simulink library "enm"  (R2022a)
settings: Solver=VariableStepAuto  StartTime=0.0  StopTime=10.0  RelTol=1e-3
undefined symbols (not defined in the file): raptor_xcp_function
libraries: Raptor_lib x7, simulink x2, slpidlib x2
settings Model: Creator=saumilj  LastModifiedBy=saumi

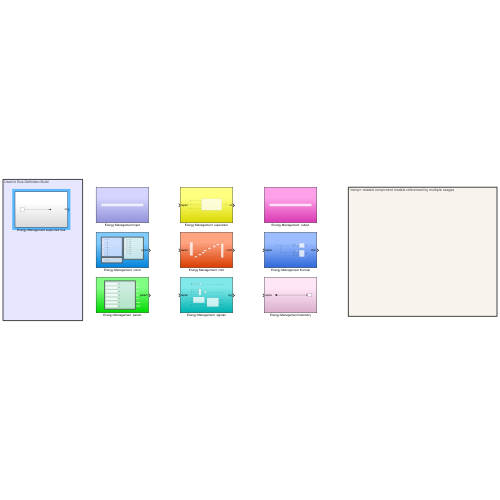
[thumbnail: Simulink's stored preview of the top-level diagram]
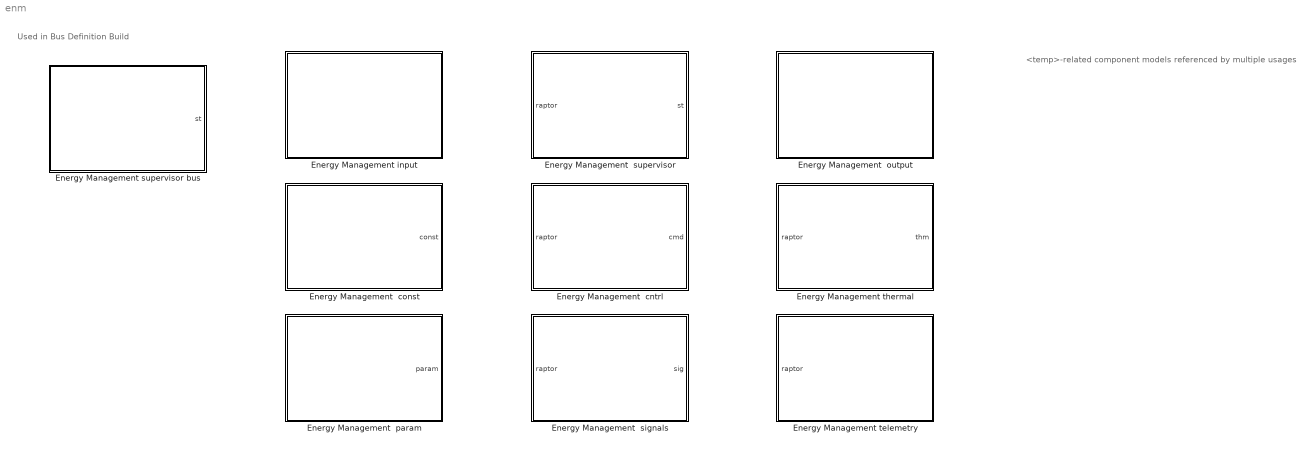
== system enm ==
  note: <temp>-related component models referenced by multiple usages
  note: Used in Bus Definition Build
  Energy Management  cntrl : Subsystem
  Energy Management  const : Subsystem
  Energy Management  output : Subsystem
  Energy Management  param : Subsystem
  Energy Management  signals : Subsystem
  Energy Management  supervisor : Subsystem
  Energy Management input : Subsystem
  Energy Management supervisor bus : Subsystem
  Energy Management telemetry : Subsystem
  Energy Management thermal : Subsystem

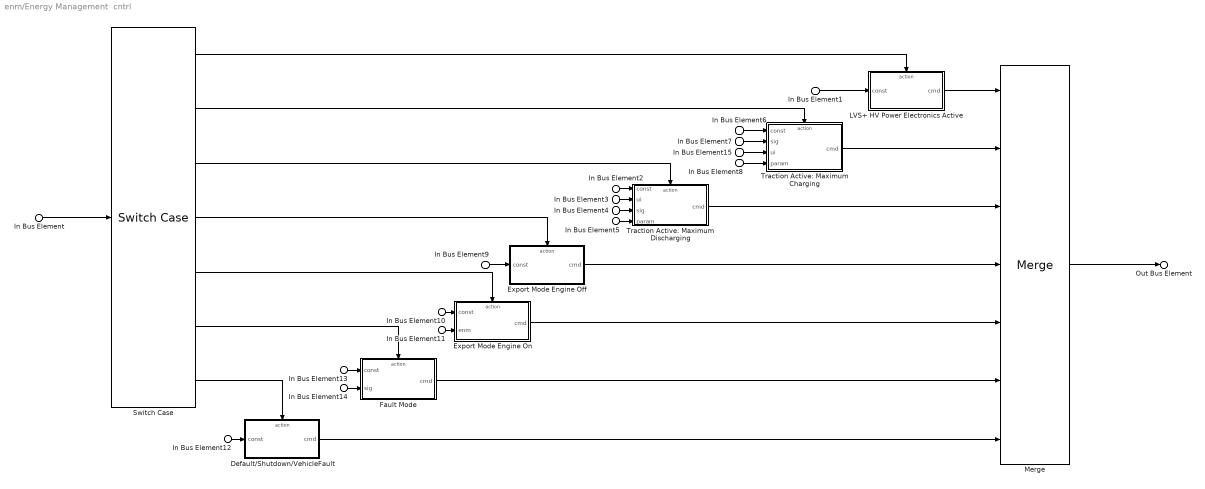
== system enm/Energy Management  cntrl ==
  In Bus Element11 : Inport  PortName=raptor  Element=enm
  In Bus Element : Inport  PortName=raptor  Element=enm.st
  In Bus Element{1..2,6,9..10,12..13} (7 alike) : Inport  PortName=raptor  Element=enm.const
  In Bus Element4 : Inport  PortName=raptor  Element=enm.sig
  In Bus Element7 : Inport  PortName=raptor  Element=enm.sig
  In Bus Element14 : Inport  PortName=raptor  Element=enm.sig
  In Bus Element8 : Inport  PortName=raptor  Element=enm.param
  In Bus Element5 : Inport  PortName=raptor  Element=enm.param
  In Bus Element3 : Inport  PortName=raptor  Element=ui
  In Bus Element15 : Inport  PortName=raptor  Element=ui
  Default/Shutdown/VehicleFault : Subsystem  TreatAsAtomicUnit=on
  Export Mode Engine Off : Subsystem  TreatAsAtomicUnit=on
  Export Mode Engine On : Subsystem  TreatAsAtomicUnit=on
  Fault Mode : Subsystem  TreatAsAtomicUnit=on
  LVS+ HV Power Electronics Active : Subsystem  TreatAsAtomicUnit=on
  Merge : Merge  Inputs=7
  Switch Case : SwitchCase  CaseConditions={1,2,3,4,5,6}
  Traction Active: Maximum Charging : Subsystem  TreatAsAtomicUnit=on
  Traction Active: Maximum Discharging : Subsystem  TreatAsAtomicUnit=on
  Out Bus Element : Outport  PortName=cmd
  wires:
  In Bus Element/1 -> Switch Case/1
  Merge/1 -> Out Bus Element/1
  Switch Case/7 -> Default/Shutdown/VehicleFault/Action
  LVS+ HV Power Electronics Active/1(cmd) -> Merge/1
  Traction Active: Maximum Charging/1(cmd) -> Merge/2
  Traction Active: Maximum Discharging/1(cmd) -> Merge/3
  Export Mode Engine Off/1(cmd) -> Merge/4
  Export Mode Engine On/1(cmd) -> Merge/5
  Fault Mode/1(cmd) -> Merge/6
  Default/Shutdown/VehicleFault/1(cmd) -> Merge/7
  Switch Case/6 -> Fault Mode/Action
  Switch Case/5 -> Export Mode Engine On/Action
  Switch Case/4 -> Export Mode Engine Off/Action
  Switch Case/3 -> Traction Active: Maximum Discharging/Action
  Switch Case/2 -> Traction Active: Maximum Charging/Action
  Switch Case/1 -> LVS+ HV Power Electronics Active/Action
  In Bus Element1/1 -> LVS+ HV Power Electronics Active/1(const)
  In Bus Element2/1 -> Traction Active: Maximum Discharging/1(const)
  In Bus Element3/1 -> Traction Active: Maximum Discharging/2(ui)
  In Bus Element4/1 -> Traction Active: Maximum Discharging/3(sig)
  In Bus Element5/1 -> Traction Active: Maximum Discharging/4(param)
  In Bus Element6/1 -> Traction Active: Maximum Charging/1(const)
  In Bus Element7/1 -> Traction Active: Maximum Charging/2(sig)
  In Bus Element8/1 -> Traction Active: Maximum Charging/4(param)
  In Bus Element9/1 -> Export Mode Engine Off/1(const)
  In Bus Element10/1 -> Export Mode Engine On/1(const)
  In Bus Element11/1 -> Export Mode Engine On/2(enm)
  In Bus Element12/1 -> Default/Shutdown/VehicleFault/1(const)
  In Bus Element13/1 -> Fault Mode/1(const)
  In Bus Element14/1 -> Fault Mode/2(sig)
  In Bus Element15/1 -> Traction Active: Maximum Charging/3(ui)

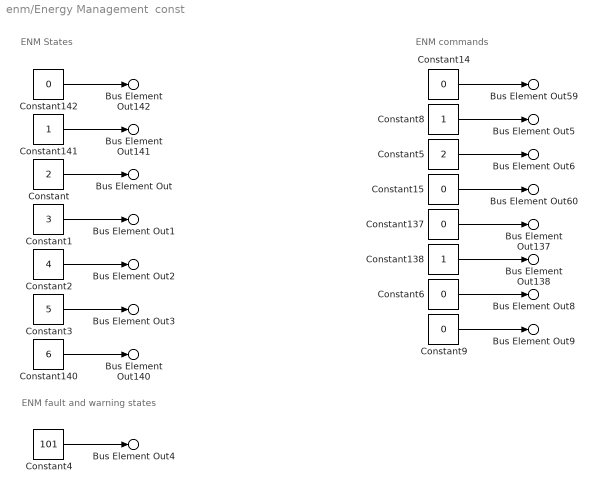
== system enm/Energy Management  const ==
  note: ENM commands
  note: ENM fault and warning states
  note: ENM States
  Constant : Constant  Value=2
  Constant1 : Constant  Value=3
  Constant{6,9,14..15,137,142} (6 alike) : Constant  Value=0
  Constant138 : Constant
  Constant140 : Constant  Value=6
  Constant141 : Constant
  Constant2 : Constant  Value=4
  Constant3 : Constant  Value=5
  Constant4 : Constant  Value=101
  Constant5 : Constant  Value=2
  Constant8 : Constant
  Bus Element Out : Outport  PortName=const  Element=ENM_2_TRACTION_ACTIVE_MAX_CHARGING
  Bus Element Out1 : Outport  PortName=const  Element=ENM_3_TRACTION_ACTIVE_MAX_DISCHARGING
  Bus Element Out2 : Outport  PortName=const  Element=ENM_4_EXPORT_ENG_OFF
  Bus Element Out3 : Outport  PortName=const  Element=ENM_5_EXPORT_ENG_ON
  Bus Element Out59 : Outport  PortName=const  Element=ENM_0_ENG_OFF
  Bus Element Out60 : Outport  PortName=const  Element=ENM_0_ENG_ZERO_POWER_DEMAND
  Bus Element Out137 : Outport  PortName=const  Element=ENM_0_TRAC_REGEN_DISABLE
  Bus Element Out138 : Outport  PortName=const  Element=ENM_1_TRAC_REGEN_ENABLE
  Bus Element Out140 : Outport  PortName=const  Element=ENM_10_SHUTDOWN
  Bus Element Out141 : Outport  PortName=const  Element=ENM_1_IDLE
  Bus Element Out142 : Outport  PortName=const  Element=ENM_0_DEFAULT
  Bus Element Out4 : Outport  PortName=const  Element=ENM_101_REDUCED_POWER
  Bus Element Out5 : Outport  PortName=const  Element=ENM_1_ENG_IDLE
  Bus Element Out6 : Outport  PortName=const  Element=ENM_2_ENG_ON
  Bus Element Out8 : Outport  PortName=const  Element=ENM_0_TRAC_ZERO_SUM_MAX_TQ
  Bus Element Out9 : Outport  PortName=const  Element=ENM_0_TRAC_ZERO_SUM_MIN_TQ
  wires:
  Constant14/1 -> Bus Element Out59/1
  Constant1/1 -> Bus Element Out1/1
  Constant140/1 -> Bus Element Out140/1
  Constant142/1 -> Bus Element Out142/1
  Constant141/1 -> Bus Element Out141/1
  Constant4/1 -> Bus Element Out4/1
  Constant137/1 -> Bus Element Out137/1
  Constant138/1 -> Bus Element Out138/1
  Constant2/1 -> Bus Element Out2/1
  Constant/1 -> Bus Element Out/1
  Constant15/1 -> Bus Element Out60/1
  Constant3/1 -> Bus Element Out3/1
  Constant8/1 -> Bus Element Out5/1
  Constant5/1 -> Bus Element Out6/1
  Constant9/1 -> Bus Element Out9/1
  Constant6/1 -> Bus Element Out8/1

== system enm/Energy Management  output ==
  note: There aren't any outputs for the Energy Management

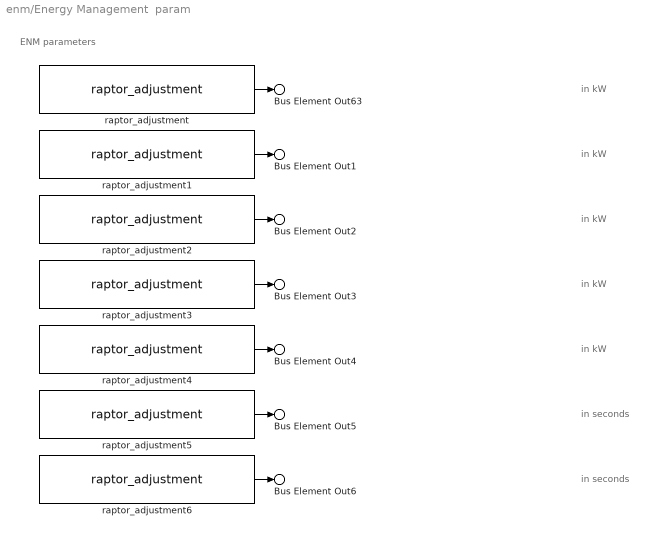
== system enm/Energy Management  param ==
  note: in kW
  note: ENM parameters
  note: in kW
  note: in kW
  note: in kW
  note: in kW
  note: in seconds
  note: in seconds
  raptor_adjustment : Raptor_lib/Data Storage/raptor_adjustment  paramName='enm_eng_max_power'  nameSource=Parameter  initValue=0  dataType=double  storage=Calibration  calDispType=Number  calEnum={'False', 'True'}  calGain=1.0  calOffset=0.0  calMax=120  calMin=0  calFormat='-1'  calUnit='kW'  calHelp='High Voltage Battery timeout in seconds'  calAccess=1  calFunction=raptor_xcp_function(gcb)  calDispHeaders=off  calColHeaders={'Col1' 'Col2' 'Col3'}  calRowHeaders={'Row1' 'Row2' 'Row3'}
      settings: SourceProductName=Raptor
  raptor_adjustment1 : Raptor_lib/Data Storage/raptor_adjustment  paramName='enm_min_hvb_power_nominal'  nameSource=Parameter  initValue=0  dataType=double  storage=Calibration  calDispType=Number  calEnum={'False', 'True'}  calGain=1.0  calOffset=0.0  calMax=120  calMin=0  calFormat='-1'  calUnit='kW'  calHelp='High Voltage Battery timeout in seconds'  calAccess=1  calFunction=raptor_xcp_function(gcb)  calDispHeaders=off  calColHeaders={'Col1' 'Col2' 'Col3'}  calRowHeaders={'Row1' 'Row2' 'Row3'}
      settings: SourceProductName=Raptor
  raptor_adjustment2 : Raptor_lib/Data Storage/raptor_adjustment  paramName='enm_max_hvb_power_nominal'  nameSource=Parameter  initValue=0  dataType=double  storage=Calibration  calDispType=Number  calEnum={'False', 'True'}  calGain=1.0  calOffset=0.0  calMax=120  calMin=0  calFormat='-1'  calUnit='kW'  calHelp='High Voltage Battery timeout in seconds'  calAccess=1  calFunction=raptor_xcp_function(gcb)  calDispHeaders=off  calColHeaders={'Col1' 'Col2' 'Col3'}  calRowHeaders={'Row1' 'Row2' 'Row3'}
      settings: SourceProductName=Raptor
  raptor_adjustment3 : Raptor_lib/Data Storage/raptor_adjustment  paramName='enm_min_hvb_power_cooldown'  nameSource=Parameter  initValue=0  dataType=double  storage=Calibration  calDispType=Number  calEnum={'False', 'True'}  calGain=1.0  calOffset=0.0  calMax=120  calMin=0  calFormat='-1'  calUnit='kW'  calHelp='High Voltage Battery timeout in seconds'  calAccess=1  calFunction=raptor_xcp_function(gcb)  calDispHeaders=off  calColHeaders={'Col1' 'Col2' 'Col3'}  calRowHeaders={'Row1' 'Row2' 'Row3'}
      settings: SourceProductName=Raptor
  raptor_adjustment4 : Raptor_lib/Data Storage/raptor_adjustment  paramName='enm_max_hvb_power_cooldown'  nameSource=Parameter  initValue=0  dataType=double  storage=Calibration  calDispType=Number  calEnum={'False', 'True'}  calGain=1.0  calOffset=0.0  calMax=120  calMin=0  calFormat='-1'  calUnit='kW'  calHelp='High Voltage Battery timeout in seconds'  calAccess=1  calFunction=raptor_xcp_function(gcb)  calDispHeaders=off  calColHeaders={'Col1' 'Col2' 'Col3'}  calRowHeaders={'Row1' 'Row2' 'Row3'}
      settings: SourceProductName=Raptor
  raptor_adjustment5 : Raptor_lib/Data Storage/raptor_adjustment  paramName='enm_veh_pwr_surplus_duration_thresh'  nameSource=Parameter  initValue=0  dataType=double  storage=Calibration  calDispType=Number  calEnum={'False', 'True'}  calGain=1.0  calOffset=0.0  calMax=120  calMin=0  calFormat='-1'  calUnit='s'  calHelp='High Voltage Battery timeout in seconds'  calAccess=1  calFunction=raptor_xcp_function(gcb)  calDispHeaders=off  calColHeaders={'Col1' 'Col2' 'Col3'}  calRowHeaders={'Row1' 'Row2' 'Row3'}
      settings: SourceProductName=Raptor
  raptor_adjustment6 : Raptor_lib/Data Storage/raptor_adjustment  paramName='enm_veh_pwr_surplus_duration_thresh'  nameSource=Parameter  initValue=0  dataType=double  storage=Calibration  calDispType=Number  calEnum={'False', 'True'}  calGain=1.0  calOffset=0.0  calMax=120  calMin=0  calFormat='-1'  calUnit='s'  calHelp='High Voltage Battery timeout in seconds'  calAccess=1  calFunction=raptor_xcp_function(gcb)  calDispHeaders=off  calColHeaders={'Col1' 'Col2' 'Col3'}  calRowHeaders={'Row1' 'Row2' 'Row3'}
      settings: SourceProductName=Raptor
  Bus Element Out63 : Outport  PortName=param  Element=ENM_ENG_MAX_POWER
  Bus Element Out1 : Outport  PortName=param  Element=ENM_MIN_HVB_POWER_NOMINAL
  Bus Element Out2 : Outport  PortName=param  Element=ENM_MAX_HVB_POWER_NOMINAL
  Bus Element Out3 : Outport  PortName=param  Element=ENM_MIN_HVB_POWER_COOLDOWN
  Bus Element Out4 : Outport  PortName=param  Element=ENM_MAX_HVB_POWER_COOLDOWN
  Bus Element Out5 : Outport  PortName=param  Element=ENM_VEH_PWR_SURPLUS_DURATION_THRESH
  Bus Element Out6 : Outport  PortName=param  Element=ENM_VEH_PWR_EXCEED_DURATION_THRESH
  wires:
  raptor_adjustment/1 -> Bus Element Out63/1
  raptor_adjustment1/1 -> Bus Element Out1/1
  raptor_adjustment3/1 -> Bus Element Out3/1
  raptor_adjustment2/1 -> Bus Element Out2/1
  raptor_adjustment4/1 -> Bus Element Out4/1
  raptor_adjustment6/1 -> Bus Element Out6/1
  raptor_adjustment5/1 -> Bus Element Out5/1

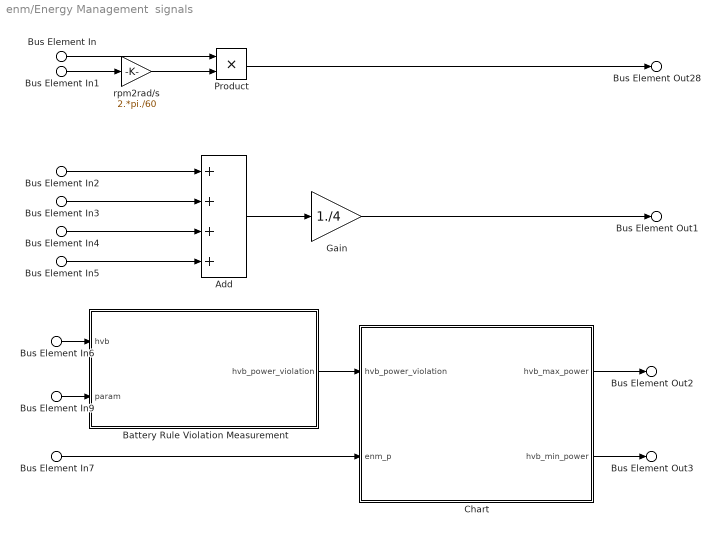
== system enm/Energy Management  signals ==
  Bus Element In : Inport  PortName=raptor  Element=gen.inp.gen_tq
  Bus Element In1 : Inport  PortName=raptor  Element=gen.inp.gen_rpm
  Bus Element In2 : Inport  PortName=raptor  Element=trac.mot1_rpm
  Bus Element In3 : Inport  PortName=raptor  Element=trac.mot2_rpm
  Bus Element In4 : Inport  PortName=raptor  Element=trac.mot3_rpm
  Bus Element In5 : Inport  PortName=raptor  Element=trac.mot4_rpm
  Bus Element In6 : Inport  PortName=raptor  Element=hvb
  Bus Element In9 : Inport  PortName=raptor  Element=enm.param
  Bus Element In7 : Inport  PortName=raptor  Element=enm.param
  Add : Sum  Inputs=++++
  "Battery Rule Violation Measurement " : Subsystem
  Chart : Stateflow chart  TreatAsAtomicUnit=on
  Gain : Gain  Gain=1./4
  Product : Product
  rpm2rad/s : Gain  Gain=2.*pi./60
  Bus Element Out28 : Outport  PortName=sig  Element=generator_power
  Bus Element Out1 : Outport  PortName=sig  Element=avg_mot_rpm
  Bus Element Out2 : Outport  PortName=sig  Element=hvb_max_power
  Bus Element Out3 : Outport  PortName=sig  Element=hvb_min_power
  wires:
  Product/1 -> Bus Element Out28/1
  Bus Element In/1 -> Product/1
  Bus Element In1/1 -> rpm2rad/s/1
  rpm2rad/s/1 -> Product/2
  Bus Element In2/1 -> Add/1
  Bus Element In3/1 -> Add/2
  Bus Element In4/1 -> Add/3
  Bus Element In5/1 -> Add/4
  Add/1 -> Gain/1
  Gain/1 -> Bus Element Out1/1
  Bus Element In6/1 -> "Battery Rule Violation Measurement "/1(hvb)
  Bus Element In9/1 -> "Battery Rule Violation Measurement "/2(param)
  "Battery Rule Violation Measurement "/1(hvb_power_violation) -> Chart/1(hvb_power_violation)
  Bus Element In7/1 -> Chart/2(enm_p)
  Chart/1(hvb_max_power) -> Bus Element Out2/1
  Chart/2(hvb_min_power) -> Bus Element Out3/1

== system enm/Energy Management  supervisor ==
  In Bus Element : Inport  PortName=raptor  Element=hvb.inp.SOC
  In Bus Element1 : Inport  PortName=raptor  Element=vss.st
  In Bus Element2 : Inport  PortName=raptor  Element=enm.const
  Energy Management Supervisor : Stateflow chart  TreatAsAtomicUnit=on
  Out Bus Element : Outport  PortName=st
  wires:
  Energy Management Supervisor/1(st) -> Out Bus Element/1
  In Bus Element/1 -> Energy Management Supervisor/1(hvb_soc)
  In Bus Element1/1 -> Energy Management Supervisor/2(sysSt)
  In Bus Element2/1 -> Energy Management Supervisor/3(c)

== system enm/Energy Management input ==
  note: There aren't any inputs for the Energy Management

== system enm/Energy Management supervisor bus ==
  Constant : Constant  Value=0
  Out Bus Element : Outport  PortName=st  Element=enmSt
  wires:
  Constant/1 -> Out Bus Element/1

== system enm/Energy Management telemetry ==
  Bus Element In : Inport  PortName=raptor
  Terminator : Terminator
  wires:
  Bus Element In/1 -> Terminator/1

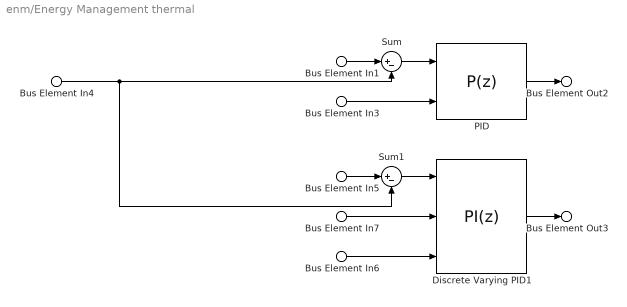
== system enm/Energy Management thermal ==
  Bus Element In1 : Inport  PortName=raptor  Element=param.<LIBNAME>_PMP_T_TARGET
  Bus Element In3 : Inport  PortName=raptor  Element=param.<LIBNAME>_PMP_PGAIN
  Bus Element In5 : Inport  PortName=raptor  Element=param.<LIBNAME>_FAN_T_TARGET
  Bus Element In7 : Inport  PortName=raptor  Element=param.<LIBNAME>_FAN_PGAIN
  Bus Element In6 : Inport  PortName=raptor  Element=param.<LIBNAME>_FAN_IGAIN
  Bus Element In4 : Inport  PortName=raptor  Element=sig.libname_temp
  " PID" : slpidlib/PID Controller  Controller=P  Form=Parallel  TimeDomain=Discrete-time  UseExternalTs=off  SampleTime=-1  IntegratorMethod=Forward Euler  FilterMethod=Forward Euler  ControllerParametersSource=external  P=1  I=1  UseKiTs=off  D=0  N=100  UseFilter=on  TunerSelectOption=Transfer Function Based (PID Tuner App)  InitialConditionSource=internal  InitialConditionForIntegrator=0  InitialConditionForFilter=0  DifferentiatorICPrevScaledInput=0  ExternalReset=none  TrackingMode=off  Kt=1  LimitOutput=on  SatLimitsSource=internal  UpperSaturationLimit=1  LowerSaturationLimit=0  LinearizeAsGain=on  AntiWindupMode=clamping  Kb=1  POutMin=[]  POutMax=[]  IOutMin=[]  IOutMax=[]  DOutMin=[]  DOutMax=[]  NOutMin=[]  NOutMax=[]  SumOutMin=[]  SumOutMax=[]  SaturationOutMin=[]  SaturationOutMax=[]  PParamMin=[]  PParamMax=[]  IParamMin=[]  IParamMax=[]  DParamMin=[]  DParamMax=[]  NParamMin=[]  NParamMax=[]  KbParamMin=[]  KbParamMax=[]  KtParamMin=[]  KtParamMax=[]  KbOutMin=[]  KbOutMax=[]  KtOutMin=[]  KtOutMax=[]  IntegratorOutMin=[]  IntegratorOutMax=[]  FilterOutMin=[]  FilterOutMax=[]  SumI1OutMin=[]  SumI1OutMax=[]  SumI2OutMin=[]  SumI2OutMax=[]  SumI3OutMin=[]  SumI3OutMax=[]  SumI4OutMin=[]  SumI4OutMax=[]  SumDOutMin=[]  SumDOutMax=[]  DifferentiatorOutMin=[]  DifferentiatorOutMax=[]  FilterDiffOutCoefMin=[]  FilterDiffOutCoefMax=[]  ReciprocalOutMin=[]  ReciprocalOutMax=[]  SumDenOutMin=[]  SumDenOutMax=[]  SumNumOutMin=[]  SumNumOutMax=[]  DivideOutMin=[]  DivideOutMax=[]  UdiffTsProdOutMin=[]  UdiffTsProdOutMax=[]  NTsProdOutMin=[]  NTsProdOutMax=[]  UintegralTsProdOutMin=[]  UintegralTsProdOutMax=[]  UngainTsProdOutMin=[]  UngainTsProdOutMax=[]  ClampingZeroOutDataTypeStr=Inherit: Inherit via back propagation  ClampingZeroOutMin=[]  ClampingZeroOutMax=[]  FilterDenConstantOutDataTypeStr=Inherit: Inherit via back propagation  FilterDenConstantOutMin=[]  FilterDenConstantOutMax=[]  PCopyOutDataTypeStr=Inherit: Inherit via back propagation  PCopyOutMin=[]  PCopyOutMax=[]  NCopyOutDataTypeStr=Inherit: Inherit via back propagation  NCopyOutMin=[]  NCopyOutMax=[]  IntegratorContinuousStateAttributes=''  IntegratorStateMustResolveToSignalObject=off  IntegratorRTWStateStorageClass=Auto  FilterContinuousStateAttributes=''  FilterStateMustResolveToSignalObject=off  FilterRTWStateStorageClass=Auto  ParallelPVariant=ExternalParameters  IdealPVariant=Disabled  IVariant=Disabled  DVariant=Disabled  IntegratorVariant=Disabled  SatVariant=Enabled  AWVariant=Disabled  PCopyVariant=Disabled  TRVariant=Disabled  FdbkBlocksVariant=Forward  IdealPFdbkVariant=Disabled  SatFdbkVariant=Disabled  DerivativeFilterVariant=Disabled  NVariant=Disabled  NCopyVariant=Disabled_SignalSpec  FilterICVariant=Disabled  IntegratorICVariant=Disabled  ExternalResetVariant=Disabled  TRSumVariant=Passthrough  SumFdbkVariant=Disabled  SumVariant=Passthrough_P  TsampFilterVariant=InternalTs  TsampNgainVariant=Passthrough  TsampIntegralVariant=Disabled_SignalSpec  ExternalSaturationOutDataTypeStr=Inherit: Same as second input  aMode=0
  Discrete Varying PID1 : slpidlib/PID Controller  Controller=PI  Form=Parallel  TimeDomain=Discrete-time  UseExternalTs=off  SampleTime=-1  IntegratorMethod=Forward Euler  FilterMethod=Forward Euler  ControllerParametersSource=external  P=1  I=1  UseKiTs=off  D=0  N=100  UseFilter=on  TunerSelectOption=Transfer Function Based (PID Tuner App)  InitialConditionSource=internal  InitialConditionForIntegrator=0  InitialConditionForFilter=0  DifferentiatorICPrevScaledInput=0  ExternalReset=none  TrackingMode=off  Kt=1  LimitOutput=on  SatLimitsSource=internal  UpperSaturationLimit=1  LowerSaturationLimit=0  LinearizeAsGain=on  AntiWindupMode=clamping  Kb=1  POutMin=[]  POutMax=[]  IOutMin=[]  IOutMax=[]  DOutMin=[]  DOutMax=[]  NOutMin=[]  NOutMax=[]  SumOutMin=[]  SumOutMax=[]  SaturationOutMin=[]  SaturationOutMax=[]  PParamMin=[]  PParamMax=[]  IParamMin=[]  IParamMax=[]  DParamMin=[]  DParamMax=[]  NParamMin=[]  NParamMax=[]  KbParamMin=[]  KbParamMax=[]  KtParamMin=[]  KtParamMax=[]  KbOutMin=[]  KbOutMax=[]  KtOutMin=[]  KtOutMax=[]  IntegratorOutMin=[]  IntegratorOutMax=[]  FilterOutMin=[]  FilterOutMax=[]  SumI1OutMin=[]  SumI1OutMax=[]  SumI2OutMin=[]  SumI2OutMax=[]  SumI3OutMin=[]  SumI3OutMax=[]  SumI4OutMin=[]  SumI4OutMax=[]  SumDOutMin=[]  SumDOutMax=[]  DifferentiatorOutMin=[]  DifferentiatorOutMax=[]  FilterDiffOutCoefMin=[]  FilterDiffOutCoefMax=[]  ReciprocalOutMin=[]  ReciprocalOutMax=[]  SumDenOutMin=[]  SumDenOutMax=[]  SumNumOutMin=[]  SumNumOutMax=[]  DivideOutMin=[]  DivideOutMax=[]  UdiffTsProdOutMin=[]  UdiffTsProdOutMax=[]  NTsProdOutMin=[]  NTsProdOutMax=[]  UintegralTsProdOutMin=[]  UintegralTsProdOutMax=[]  UngainTsProdOutMin=[]  UngainTsProdOutMax=[]  ClampingZeroOutDataTypeStr=Inherit: Inherit via back propagation  ClampingZeroOutMin=[]  ClampingZeroOutMax=[]  FilterDenConstantOutDataTypeStr=Inherit: Inherit via back propagation  FilterDenConstantOutMin=[]  FilterDenConstantOutMax=[]  PCopyOutDataTypeStr=Inherit: Inherit via back propagation  PCopyOutMin=[]  PCopyOutMax=[]  NCopyOutDataTypeStr=Inherit: Inherit via back propagation  NCopyOutMin=[]  NCopyOutMax=[]  IntegratorContinuousStateAttributes=''  IntegratorStateMustResolveToSignalObject=off  IntegratorRTWStateStorageClass=Auto  FilterContinuousStateAttributes=''  FilterStateMustResolveToSignalObject=off  FilterRTWStateStorageClass=Auto  ParallelPVariant=ExternalParameters  IdealPVariant=Disabled  IVariant=ExternalParameters  DVariant=Disabled  IntegratorVariant=Discrete  SatVariant=Enabled  AWVariant=DiscClampingParallel  PCopyVariant=Disabled  TRVariant=Disabled  FdbkBlocksVariant=Forward  IdealPFdbkVariant=Disabled  SatFdbkVariant=Disabled  DerivativeFilterVariant=Disabled  NVariant=Disabled  NCopyVariant=Disabled_SignalSpec  FilterICVariant=Disabled  IntegratorICVariant=InternalICs  ExternalResetVariant=Disabled  TRSumVariant=Passthrough  SumFdbkVariant=Disabled  SumVariant=Sum_PI  TsampFilterVariant=InternalTs  TsampNgainVariant=Passthrough  TsampIntegralVariant=Passthrough  ExternalSaturationOutDataTypeStr=Inherit: Same as second input  aMode=0
  Sum : Sum  Inputs=|+-
  Sum1 : Sum  Inputs=|+-
  Bus Element Out2 : Outport  PortName=thm  Element=pmp_effort
  Bus Element Out3 : Outport  PortName=thm  Element=fan_effort
  wires:
  Bus Element In4/1 -> Sum/2, Sum1/2
  Bus Element In6/1 -> Discrete Varying PID1/3
  Bus Element In7/1 -> Discrete Varying PID1/2
  Sum/1 -> " PID"/1
  Discrete Varying PID1/1 -> Bus Element Out3/1
  Sum1/1 -> Discrete Varying PID1/1
  Bus Element In1/1 -> Sum/1
  " PID"/1 -> Bus Element Out2/1
  Bus Element In5/1 -> Sum1/1
  Bus Element In3/1 -> " PID"/2

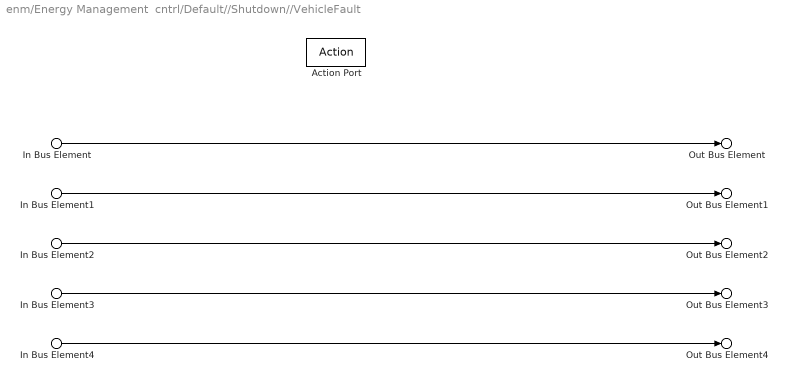
== system enm/Energy Management  cntrl/Default//Shutdown//VehicleFault ==
  In Bus Element : Inport  PortName=const  Element=ENM_0_ENG_OFF
  In Bus Element1 : Inport  PortName=const  Element=ENM_0_ENG_ZERO_POWER_DEMAND
  In Bus Element2 : Inport  PortName=const  Element=ENM_0_TRAC_REGEN_DISABLE
  In Bus Element3 : Inport  PortName=const  Element=ENM_0_TRAC_ZERO_SUM_MAX_TQ
  In Bus Element4 : Inport  PortName=const  Element=ENM_0_TRAC_ZERO_SUM_MIN_TQ
  Action Port : ActionPort  ActionPortLabel=default:
  Out Bus Element : Outport  PortName=cmd  Element=eng_state_request
  Out Bus Element1 : Outport  PortName=cmd  Element=eng_power_demand
  Out Bus Element2 : Outport  PortName=cmd  Element=trac_regen_mode
  Out Bus Element3 : Outport  PortName=cmd  Element=trac_sum_max_tq
  Out Bus Element4 : Outport  PortName=cmd  Element=trac_sum_min_tq
  wires:
  In Bus Element2/1 -> Out Bus Element2/1
  In Bus Element4/1 -> Out Bus Element4/1
  In Bus Element3/1 -> Out Bus Element3/1
  In Bus Element/1 -> Out Bus Element/1
  In Bus Element1/1 -> Out Bus Element1/1

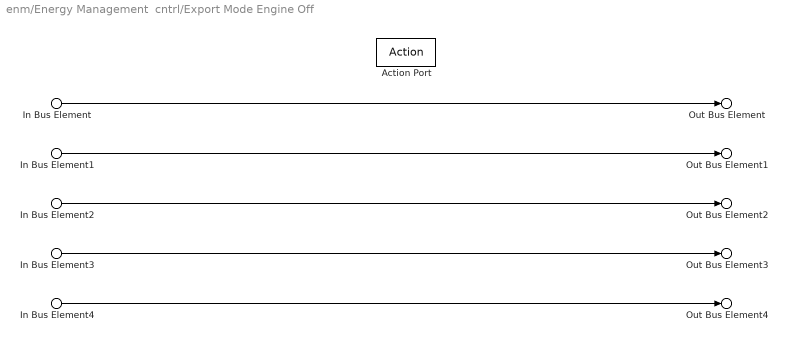
== system enm/Energy Management  cntrl/Export Mode Engine Off ==
  In Bus Element : Inport  PortName=const  Element=ENM_0_ENG_OFF
  In Bus Element1 : Inport  PortName=const  Element=ENM_0_ENG_ZERO_POWER_DEMAND
  In Bus Element2 : Inport  PortName=const  Element=ENM_0_TRAC_REGEN_DISABLE
  In Bus Element3 : Inport  PortName=const  Element=ENM_0_TRAC_ZERO_SUM_MAX_TQ
  In Bus Element4 : Inport  PortName=const  Element=ENM_0_TRAC_ZERO_SUM_MIN_TQ
  Action Port : ActionPort  ActionPortLabel=case [ 4 ]:
  Out Bus Element : Outport  PortName=cmd  Element=eng_state_request
  Out Bus Element1 : Outport  PortName=cmd  Element=eng_power_demand
  Out Bus Element2 : Outport  PortName=cmd  Element=trac_regen_mode
  Out Bus Element3 : Outport  PortName=cmd  Element=trac_sum_max_tq
  Out Bus Element4 : Outport  PortName=cmd  Element=trac_sum_min_tq
  wires:
  In Bus Element2/1 -> Out Bus Element2/1
  In Bus Element4/1 -> Out Bus Element4/1
  In Bus Element3/1 -> Out Bus Element3/1
  In Bus Element/1 -> Out Bus Element/1
  In Bus Element1/1 -> Out Bus Element1/1

== system enm/Energy Management  cntrl/Export Mode Engine On ==
  In Bus Element : Inport  PortName=const  Element=ENM_0_ENG_OFF
  In Bus Element2 : Inport  PortName=const  Element=ENM_0_TRAC_REGEN_DISABLE
  In Bus Element3 : Inport  PortName=const  Element=ENM_0_TRAC_ZERO_SUM_MAX_TQ
  In Bus Element4 : Inport  PortName=const  Element=ENM_0_TRAC_ZERO_SUM_MIN_TQ
  In Bus Element6 : Inport  Port=2  PortName=enm  Element=param.ENM_ENG_MAX_POWER
  Action Port : ActionPort  ActionPortLabel=case [ 5 ]:
  Out Bus Element : Outport  PortName=cmd  Element=eng_state_request
  Out Bus Element1 : Outport  PortName=cmd  Element=eng_power_demand
  Out Bus Element2 : Outport  PortName=cmd  Element=trac_regen_mode
  Out Bus Element3 : Outport  PortName=cmd  Element=trac_sum_max_tq
  Out Bus Element4 : Outport  PortName=cmd  Element=trac_sum_min_tq
  wires:
  In Bus Element/1 -> Out Bus Element/1
  In Bus Element6/1 -> Out Bus Element1/1
  In Bus Element3/1 -> Out Bus Element3/1
  In Bus Element4/1 -> Out Bus Element4/1
  In Bus Element2/1 -> Out Bus Element2/1

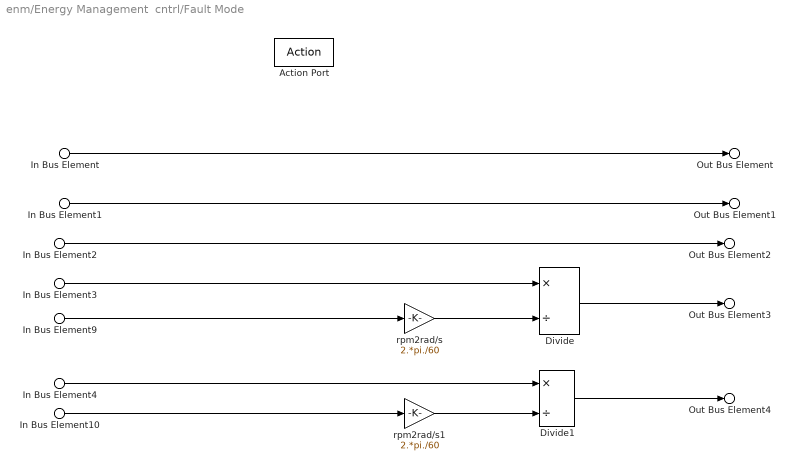
== system enm/Energy Management  cntrl/Fault Mode ==
  In Bus Element2 : Inport  PortName=const  Element=ENM_1_TRAC_REGEN_ENABLE
  In Bus Element : Inport  PortName=const  Element=ENM_0_ENG_OFF
  In Bus Element1 : Inport  PortName=const  Element=ENM_0_ENG_ZERO_POWER_DEMAND
  In Bus Element3 : Inport  Port=2  PortName=sig  Element=max_hvb_power
  In Bus Element9 : Inport  Port=2  PortName=sig  Element=avg_mot_rpm
  In Bus Element10 : Inport  Port=2  PortName=sig  Element=avg_mot_rpm
  In Bus Element4 : Inport  Port=2  PortName=sig  Element=min_hvb_power
  Action Port : ActionPort  ActionPortLabel=case [ 6 ]:
  Divide : Product  Inputs=*/
  Divide1 : Product  Inputs=*/
  rpm2rad/s : Gain  Gain=2.*pi./60
  rpm2rad/s1 : Gain  Gain=2.*pi./60
  Out Bus Element2 : Outport  PortName=cmd  Element=trac_regen_mode
  Out Bus Element3 : Outport  PortName=cmd  Element=trac_sum_max_tq
  Out Bus Element4 : Outport  PortName=cmd  Element=trac_sum_min_tq
  Out Bus Element : Outport  PortName=cmd  Element=eng_state_request
  Out Bus Element1 : Outport  PortName=cmd  Element=eng_power_demand
  wires:
  In Bus Element2/1 -> Out Bus Element2/1
  In Bus Element3/1 -> Divide/1
  rpm2rad/s/1 -> Divide/2
  Divide/1 -> Out Bus Element3/1
  In Bus Element4/1 -> Divide1/1
  Divide1/1 -> Out Bus Element4/1
  rpm2rad/s1/1 -> Divide1/2
  In Bus Element10/1 -> rpm2rad/s1/1
  In Bus Element9/1 -> rpm2rad/s/1
  In Bus Element1/1 -> Out Bus Element1/1
  In Bus Element/1 -> Out Bus Element/1

== system enm/Energy Management  cntrl/LVS+ HV Power Electronics Active ==
  In Bus Element : Inport  PortName=const  Element=ENM_0_ENG_OFF
  In Bus Element1 : Inport  PortName=const  Element=ENM_0_ENG_ZERO_POWER_DEMAND
  In Bus Element2 : Inport  PortName=const  Element=ENM_0_TRAC_REGEN_DISABLE
  In Bus Element3 : Inport  PortName=const  Element=ENM_0_TRAC_ZERO_SUM_MAX_TQ
  In Bus Element4 : Inport  PortName=const  Element=ENM_0_TRAC_ZERO_SUM_MIN_TQ
  Action Port : ActionPort  ActionPortLabel=case [ 1 ]:
  Out Bus Element : Outport  PortName=cmd  Element=eng_state_request
  Out Bus Element1 : Outport  PortName=cmd  Element=eng_power_demand
  Out Bus Element2 : Outport  PortName=cmd  Element=trac_regen_mode
  Out Bus Element3 : Outport  PortName=cmd  Element=trac_sum_max_tq
  Out Bus Element4 : Outport  PortName=cmd  Element=trac_sum_min_tq
  wires:
  In Bus Element/1 -> Out Bus Element/1
  In Bus Element1/1 -> Out Bus Element1/1
  In Bus Element2/1 -> Out Bus Element2/1
  In Bus Element3/1 -> Out Bus Element3/1
  In Bus Element4/1 -> Out Bus Element4/1

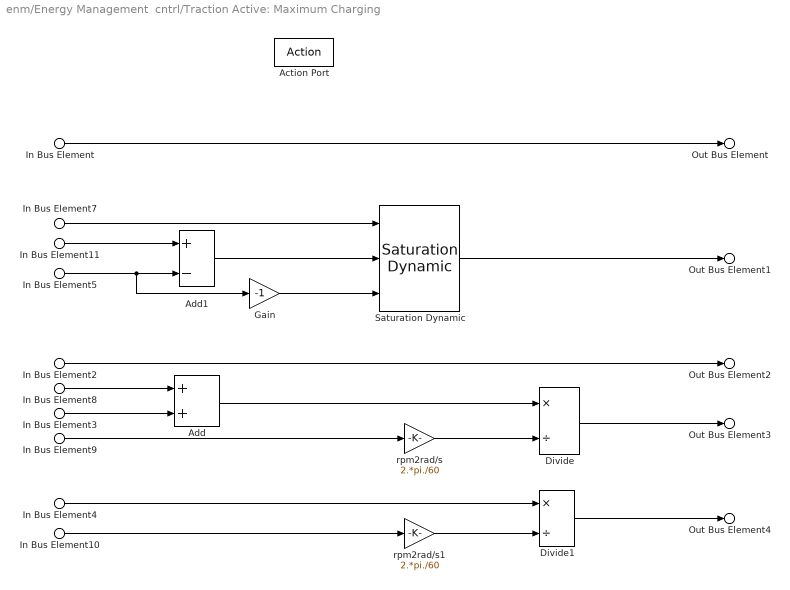
== system enm/Energy Management  cntrl/Traction Active: Maximum Charging ==
  In Bus Element : Inport  PortName=const  Element=ENM_2_ENG_ON
  In Bus Element2 : Inport  PortName=const  Element=ENM_1_TRAC_REGEN_ENABLE
  In Bus Element3 : Inport  Port=2  PortName=sig  Element=hvb_max_power
  In Bus Element8 : Inport  Port=2  PortName=sig  Element=generator_power
  In Bus Element9 : Inport  Port=2  PortName=sig  Element=avg_mot_rpm
  In Bus Element10 : Inport  Port=2  PortName=sig  Element=avg_mot_rpm
  In Bus Element5 : Inport  Port=2  PortName=sig  Element=hvb_min_power
  In Bus Element4 : Inport  Port=2  PortName=sig  Element=hvb_min_power
  In Bus Element11 : Inport  Port=3  PortName=ui  Element=sig.veh_power_demand
  In Bus Element7 : Inport  Port=4  PortName=param  Element=ENM_ENG_MAX_POWER
  Action Port : ActionPort  ActionPortLabel=case [ 2 ]:
  Add : Sum
  Add1 : Sum  Inputs=+-
  Divide : Product  Inputs=*/
  Divide1 : Product  Inputs=*/
  Gain : Gain  Gain=-1
  Saturation Dynamic : simulink/Discontinuities/Saturation Dynamic  OutMin=[]  OutMax=[]  OutDataTypeStr=Inherit: Same as second input  OutDataType=fixdt(1, 16)  OutScaling=2^-10  DoSatur=off
  rpm2rad/s : Gain  Gain=2.*pi./60
  rpm2rad/s1 : Gain  Gain=2.*pi./60
  Out Bus Element : Outport  PortName=cmd  Element=eng_state_request
  Out Bus Element1 : Outport  PortName=cmd  Element=eng_power_demand
  Out Bus Element2 : Outport  PortName=cmd  Element=trac_regen_mode
  Out Bus Element3 : Outport  PortName=cmd  Element=trac_sum_max_tq
  Out Bus Element4 : Outport  PortName=cmd  Element=trac_sum_min_tq
  wires:
  In Bus Element9/1 -> rpm2rad/s/1
  Divide1/1 -> Out Bus Element4/1
  In Bus Element10/1 -> rpm2rad/s1/1
  In Bus Element/1 -> Out Bus Element/1
  In Bus Element8/1 -> Add/1
  rpm2rad/s1/1 -> Divide1/2
  In Bus Element4/1 -> Divide1/1
  rpm2rad/s/1 -> Divide/2
  Add/1 -> Divide/1
  In Bus Element3/1 -> Add/2
  Divide/1 -> Out Bus Element3/1
  In Bus Element2/1 -> Out Bus Element2/1
  In Bus Element5/1 -> Gain/1, Add1/2
  In Bus Element11/1 -> Add1/1
  In Bus Element7/1 -> Saturation Dynamic/1
  Gain/1 -> Saturation Dynamic/3
  Add1/1 -> Saturation Dynamic/2
  Saturation Dynamic/1 -> Out Bus Element1/1

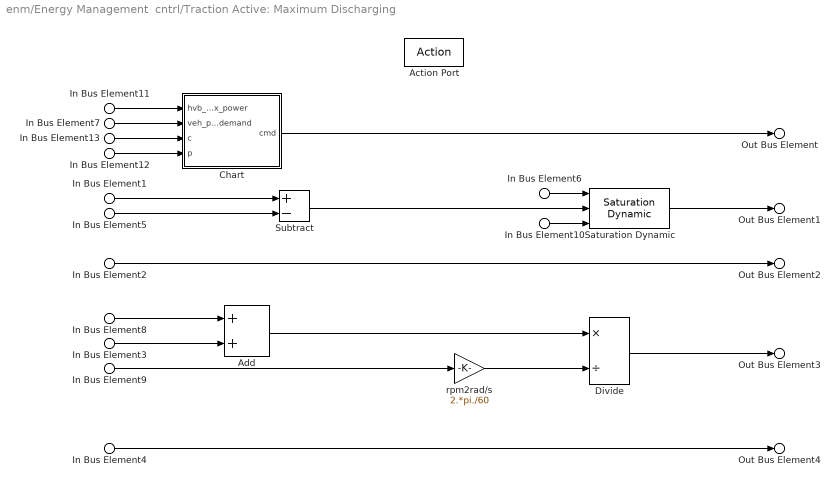
== system enm/Energy Management  cntrl/Traction Active: Maximum Discharging ==
  In Bus Element13 : Inport  PortName=const
  In Bus Element2 : Inport  PortName=const  Element=ENM_0_TRAC_REGEN_DISABLE
  In Bus Element4 : Inport  PortName=const  Element=ENM_0_TRAC_ZERO_SUM_MIN_TQ
  In Bus Element10 : Inport  PortName=const  Element=ENM_0_ENG_ZERO_POWER_DEMAND
  In Bus Element1 : Inport  Port=2  PortName=ui  Element=sig.veh_power_demand
  In Bus Element7 : Inport  Port=2  PortName=ui  Element=sig.veh_power_demand
  In Bus Element8 : Inport  Port=3  PortName=sig  Element=generator_power
  In Bus Element9 : Inport  Port=3  PortName=sig  Element=avg_mot_rpm
  In Bus Element3 : Inport  Port=3  PortName=sig  Element=hvb_max_power
  In Bus Element5 : Inport  Port=3  PortName=sig  Element=hvb_max_power
  In Bus Element11 : Inport  Port=3  PortName=sig  Element=hvb_max_power
  In Bus Element12 : Inport  Port=4  PortName=param
  In Bus Element6 : Inport  Port=4  PortName=param  Element=ENM_ENG_MAX_POWER
  Action Port : ActionPort  ActionPortLabel=case [ 3 ]:
  Add : Sum
  Chart : Stateflow chart  TreatAsAtomicUnit=on
  Divide : Product  Inputs=*/
  Saturation Dynamic : simulink/Discontinuities/Saturation Dynamic  OutMin=[]  OutMax=[]  OutDataTypeStr=Inherit: Same as second input  OutDataType=fixdt(1, 16)  OutScaling=2^-10  DoSatur=off
  Subtract : Sum  Inputs=+-
  rpm2rad/s : Gain  Gain=2.*pi./60
  Out Bus Element : Outport  PortName=cmd  Element=eng_state_request
  Out Bus Element1 : Outport  PortName=cmd  Element=eng_power_demand
  Out Bus Element2 : Outport  PortName=cmd  Element=trac_regen_mode
  Out Bus Element3 : Outport  PortName=cmd  Element=trac_sum_max_tq
  Out Bus Element4 : Outport  PortName=cmd  Element=trac_sum_min_tq
  wires:
  In Bus Element9/1 -> rpm2rad/s/1
  In Bus Element6/1 -> Saturation Dynamic/1
  Divide/1 -> Out Bus Element3/1
  In Bus Element10/1 -> Saturation Dynamic/3
  In Bus Element5/1 -> Subtract/2
  In Bus Element3/1 -> Add/2
  Saturation Dynamic/1 -> Out Bus Element1/1
  rpm2rad/s/1 -> Divide/2
  In Bus Element1/1 -> Subtract/1
  In Bus Element2/1 -> Out Bus Element2/1
  Subtract/1 -> Saturation Dynamic/2
  Add/1 -> Divide/1
  In Bus Element8/1 -> Add/1
  In Bus Element4/1 -> Out Bus Element4/1
  In Bus Element7/1 -> Chart/2(veh_power_demand)
  In Bus Element11/1 -> Chart/1(hvb_max_power)
  In Bus Element13/1 -> Chart/3(c)
  In Bus Element12/1 -> Chart/4(p)
  Chart/1(cmd) -> Out Bus Element/1

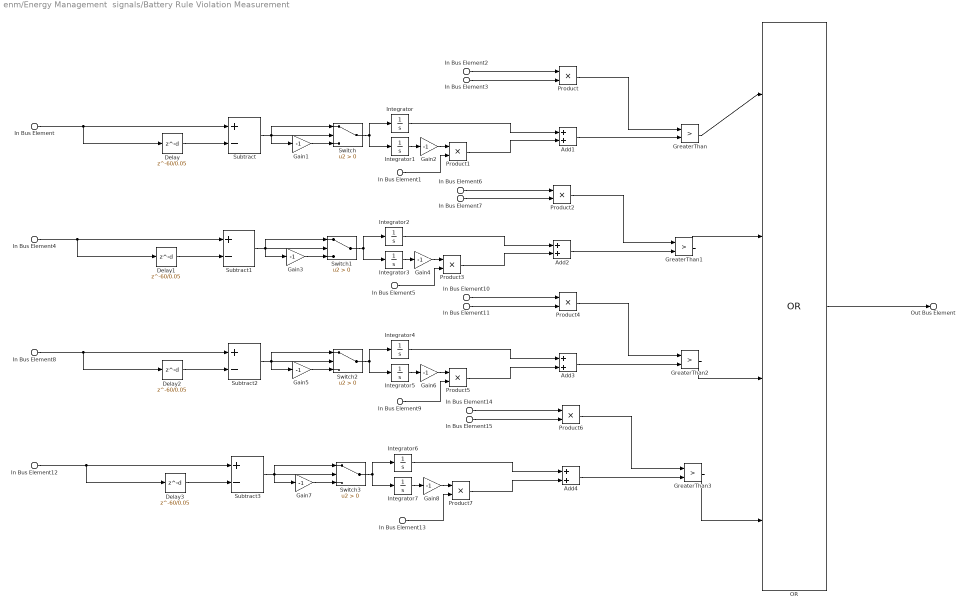
== system enm/Energy Management  signals/Battery Rule Violation Measurement  ==
  In Bus Element{,4,8,12} (4 alike) : Inport  PortName=hvb  Element=inp.power
  In Bus Element{1,5,9,13} (4 alike) : Inport  Port=2  PortName=param  Element=ENM_HVB_CHARGE_CURR_WEIGHTING
  In Bus Element{2,6,10,14} (4 alike) : Inport  Port=2  PortName=param  Element=ENM_HVB_MAX_DISCHARGE_CURR
  In Bus Element{3,7,11,15} (4 alike) : Inport  Port=2  PortName=param  Element=ENM_HVB_MAX_DISCHARGE_CURR_DURATION
  Add{1..4} (4 alike) : Sum
  Delay{,1..3} (4 alike) : Delay  DelayLength=60/0.05  SampleTime=0.05
  Gain{1..8} (8 alike) : Gain  Gain=-1
  GreaterThan{,1..3} (4 alike) : RelationalOperator  Operator=>  OutDataTypeStr=boolean  RndMeth=Simplest  InputSameDT=off
  Integrator{,1..7} (8 alike) : Integrator
  OR : Logic  Operator=OR  Inputs=4  IconShape=distinctive  AllPortsSameDT=off  OutDataTypeStr=boolean
  Product{,1..7} (8 alike) : Product
  Subtract{,1..3} (4 alike) : Sum  Inputs=+-
  Switch{,1..3} (4 alike) : Switch  Criteria=u2 > Threshold  SaturateOnIntegerOverflow=off  InputSameDT=off
  Out Bus Element : Outport  PortName=hvb_power_violation
  wires:
  Gain1/1 -> Switch/3
  Subtract/1 -> Switch/1, Gain1/1, Switch/2
  Gain2/1 -> Product1/1
  Integrator/1 -> Add1/1
  Switch/1 -> Integrator1/1, Integrator/1
  Product1/1 -> Add1/2
  Delay/1 -> Subtract/2
  Integrator1/1 -> Gain2/1
  In Bus Element/1 -> Delay/1, Subtract/1
  In Bus Element1/1 -> Product1/2
  In Bus Element2/1 -> Product/1
  In Bus Element3/1 -> Product/2
  Add1/1 -> GreaterThan/2
  Product/1 -> GreaterThan/1
  GreaterThan/1 -> OR/1
  Product2/1 -> GreaterThan1/1
  Add2/1 -> GreaterThan1/2
  In Bus Element7/1 -> Product2/2
  In Bus Element6/1 -> Product2/1
  In Bus Element5/1 -> Product3/2
  In Bus Element4/1 -> Subtract1/1, Delay1/1
  Integrator3/1 -> Gain4/1
  Delay1/1 -> Subtract1/2
  Product3/1 -> Add2/2
  Switch1/1 -> Integrator2/1, Integrator3/1
  Integrator2/1 -> Add2/1
  Gain4/1 -> Product3/1
  Subtract1/1 -> Switch1/2, Gain3/1, Switch1/1
  Gain3/1 -> Switch1/3
  Gain5/1 -> Switch2/3
  Subtract2/1 -> Switch2/1, Gain5/1, Switch2/2
  Gain6/1 -> Product5/1
  Integrator4/1 -> Add3/1
  Switch2/1 -> Integrator5/1, Integrator4/1
  Product5/1 -> Add3/2
  Delay2/1 -> Subtract2/2
  Integrator5/1 -> Gain6/1
  In Bus Element8/1 -> Delay2/1, Subtract2/1
  In Bus Element9/1 -> Product5/2
  In Bus Element10/1 -> Product4/1
  In Bus Element11/1 -> Product4/2
  Add3/1 -> GreaterThan2/2
  Product4/1 -> GreaterThan2/1
  Product6/1 -> GreaterThan3/1
  Add4/1 -> GreaterThan3/2
  In Bus Element15/1 -> Product6/2
  In Bus Element14/1 -> Product6/1
  In Bus Element13/1 -> Product7/2
  In Bus Element12/1 -> Subtract3/1, Delay3/1
  Integrator7/1 -> Gain8/1
  Delay3/1 -> Subtract3/2
  Product7/1 -> Add4/2
  Switch3/1 -> Integrator6/1, Integrator7/1
  Integrator6/1 -> Add4/1
  Gain8/1 -> Product7/1
  Subtract3/1 -> Switch3/2, Gain7/1, Switch3/1
  Gain7/1 -> Switch3/3
  GreaterThan1/1 -> OR/2
  GreaterThan2/1 -> OR/3
  GreaterThan3/1 -> OR/4
  OR/1 -> Out Bus Element/1

== stateflow chart enm/Energy Management  cntrl/Traction Active: Maximum Discharging/Chart ==
  state engineOff
    cmd = c.ENM_0_ENG_OFF;
  state engineOn
    cmd = c.ENM_2_ENG_ON
  (default) -> engineOff
  engineOn -> engineOff : [duration(veh_power_demand > hvb_max_power) == p.ENM_VEH_PWR_SURPLUS_DURATION_THRESH]
  engineOff -> engineOn : [duration(veh_power_demand > hvb_max_power) == p.ENM_VEH_PWR_EXCEED_DURATION_THRESHOLD]
  data: hvb_max_power input; cmd output; veh_power_demand input; c input; p input

== stateflow chart enm/Energy Management  signals/Chart ==
  state nominal
    hvb_min_power = p.ENM_MIN_HVB_POWER_NOMINAL;
    hvb_max_power = p.ENM_MAX_HVB_POWER_NOMINAL;
  state cooldown
    hvb_min_power = p.ENM_MIN_HVB_POWER_COOLDOWN;
    hvb_max_power = p.ENM_MAX_HVB_POWER_COOLDOWN;
  (default) -> nominal
  nominal -> cooldown : [hvb_power_violation]
  cooldown -> nominal : after(enm_p.ENM_HVB_COOLDOWN_DURATION,sec)
  data: hvb_power_violation input; enm_p input; hvb_max_power output; hvb_min_power output

== stateflow chart enm/Energy Management  supervisor/Energy Management Supervisor ==
  state default
    en,du:
    st = c.ENM_0_DEFAULT;
  state nominalOperation
    state HVPEActive
      state idle
        en,du:
        st = c.ENM_1_IDLE
      state exportActive
        state engineOff
          en,du:
          st = c.ENM_4_EXPORT_ENG_OFF
        state engineOn
          en,du:
          st = c.ENM_5_EXPORT_ENG_ON
        (default) -> engineOff
        engineOff -> engineOn : [hvb_soc<= c.HVB_LO_THRESH]
        engineOn -> engineOff [order 1] : [hvb_soc>= c.HVB_HI_THRESH]
        engineOn -> (junction 919) [order 2]
      state tractionActive
        state maximizeCharging
          en,du:
          st = c.ENM_2_MAX_CHARGING
        state maximizeDischarging
          en,du:
          st = c.ENM_3_MAX_DISCHARGING
        (default) -> maximizeCharging
        maximizeCharging -> maximizeDischarging : [hvb_soc<= c.HVB_LO_THRESH]
        maximizeDischarging -> maximizeCharging [order 1] : [hvb_soc>= c.HVB_HI_THRESH]
        maximizeDischarging -> (junction 913) [order 2]
      (default) -> idle
      idle -> (junction 897) [order 2] : [sysSt == vss_c.EXPORT_MODE]
      idle -> (junction 893) [order 1] : [sysSt == vss_c.READY_TO_DRIVE]
      (junction 897) -> exportActive
      (junction 893) -> tractionActive
      (junction 941) -> idle : [sysSt ~= vss_c.READY_TO_DRIVE]
      exportActive -> (junction 941)
      tractionActive -> (junction 941)
      (junction 919) -> (junction 913)
    (default) -> HVPEActive
  state enmFault
    state enmReducedPower
      en,du:
      st = c.ENM_6_REDUCED_POWER
  state shutdown
    en,du:
    st = c.ENM_10_SHUTDOWN;
  (default) -> default
  default -> nominalOperation : [sysSt >= vss_c.INITIALIZING]
  (junction 913) -> enmReducedPower : [engSt == eng_c.ENG_START_FAILED]
  enmReducedPower -> (junction 929)
  nominalOperation -> (junction 925)
  (junction 929) -> (junction 925)
  (junction 925) -> shutdown : [sysSt>= vss_c.SS_SHUTDOWN_REQUESTED |...
      | sysSt>= vss_c.VEH_FLT_LIMIT]
  data: hvb_soc input; st output; sysSt input; c input
